simulink model "untitledu"  (R2022b)
settings: Solver=VariableStepAuto  StartTime=0.0  StopTime=10.0  RelTol=1e-3
settings Model: Creator=admin  LastModifiedBy=admin

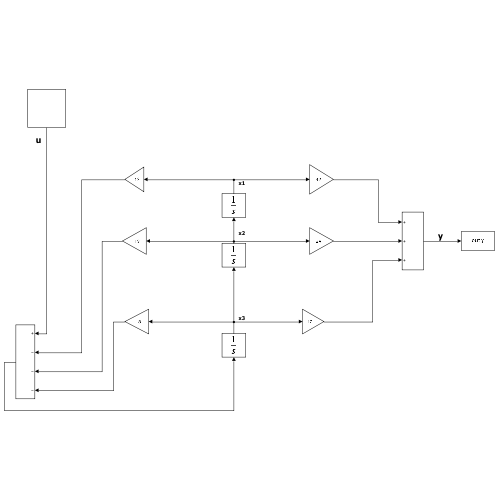
[thumbnail: Simulink's stored preview of the top-level diagram]
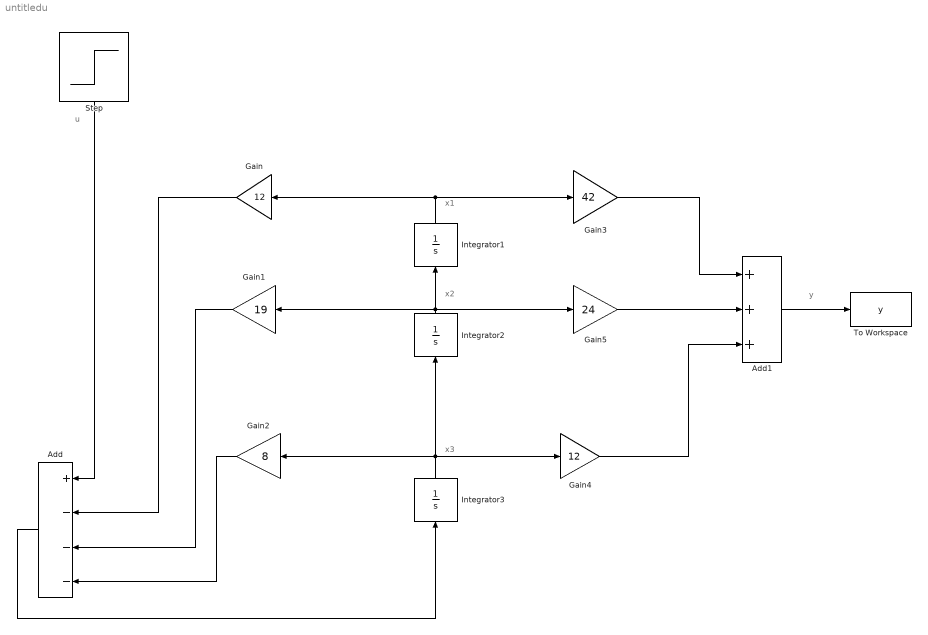
== system untitledu ==
  note: y
  note: x3
  note: x2
  note: x1
  note: u
  Add : Sum  Inputs=+---
  Add1 : Sum  Inputs=+++
  Gain : Gain  Gain=12
  Gain1 : Gain  Gain=19
  Gain2 : Gain  Gain=8
  Gain3 : Gain  Gain=42
  Gain4 : Gain  Gain=12
  Gain5 : Gain  Gain=24
  Integrator1 : Integrator
  Integrator2 : Integrator
  Integrator3 : Integrator
  Step : Step  SampleTime=0
  To Workspace : ToWorkspace  VariableName=y  SaveFormat=Structure With Time  SampleTime=-1
  wires:
  Step/1 -> Add/1
  Gain/1 -> Add/2
  Gain1/1 -> Add/3
  Gain2/1 -> Add/4
  Add/1 -> Integrator3/1
  Integrator3/1 -> Integrator2/1, Gain2/1, Gain4/1
  Integrator2/1 -> Integrator1/1, Gain1/1, Gain5/1
  Integrator1/1 -> Gain3/1, Gain/1
  Gain3/1 -> Add1/1
  Gain5/1 -> Add1/2
  Gain4/1 -> Add1/3
  Add1/1 -> To Workspace/1
